simulink model "plantmodel"  (R2020a)
settings: Solver=VariableStepAuto  StartTime=0.0  StopTime=10.0  RelTol=1e-3
undefined symbols (not defined in the file): Ax, Ay, Az, b, d, g, I, Ixx, Iyy, Izz, Jr, m
settings Model: Creator=Muni Kumar  LastModifiedBy=Muni Kumar

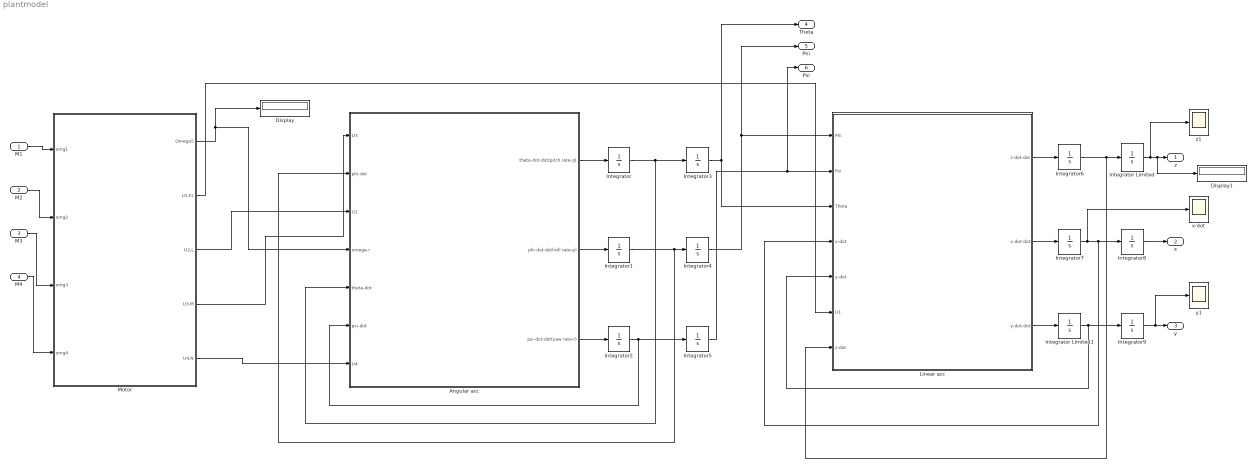
== system plantmodel ==
  M1 : Inport
  M2 : Inport  Port=2
  M3 : Inport  Port=3
  M4 : Inport  Port=4
  Angular acc : Subsystem
  Display : Display
      settings: Decimation=2
  Display1 : Display
  Integrator{,1..2,6..9} (7 alike) : Integrator
  Integrator Limited : Integrator  LimitOutput=on  UpperSaturationLimit=1  LowerSaturationLimit=0
  Integrator Limited1 : Integrator  LimitOutput=on  UpperSaturationLimit=1  LowerSaturationLimit=0
  Integrator3 : Integrator  WrapState=on
  Integrator4 : Integrator  WrapState=on
  Integrator5 : Integrator  WrapState=on
  Linear acc : Subsystem
  Motor : Subsystem
  x-dot : Scope
  y1 : Scope
  z1 : Scope
  z : Outport
  x : Outport  Port=2
  y : Outport  Port=3
  Theta : Outport  Port=4
  Phi : Outport  Port=5
  Psi : Outport  Port=6
  wires:
  Linear acc/2(x-dot-dot) -> Integrator7/1
  Integrator6/1 -> Integrator Limited/1, Linear acc/7(z-dot)
  Linear acc/1(z-dot-dot) -> Integrator6/1
  Motor/2(U1,Fz) -> Linear acc/6(U1)
  Linear acc/3(y-dot-dot) -> Integrator Limited1/1
  Integrator Limited1/1 -> Integrator9/1, Linear acc/5(y-dot)
  M3/1 -> Motor/3(omg3)
  M2/1 -> Motor/2(omg2)
  M1/1 -> Motor/1(omg1)
  M4/1 -> Motor/4(omg4)
  Angular acc/2(phi-dot-dot(roll rate-p)) -> Integrator1/1
  Angular acc/3(psi-dot-dot(yaw rate-r)) -> Integrator2/1
  Integrator/1 -> Angular acc/5(theta-dot), Integrator3/1
  Angular acc/1(theta-dot-dot(pitch rate-q)) -> Integrator/1
  Motor/5(U4,N) -> Angular acc/7(U4)
  Motor/4(U3,M) -> Angular acc/1(U3)
  Motor/3(U2,L) -> Angular acc/3(U2)
  Integrator1/1 -> Angular acc/2(phi-dot), Integrator4/1
  Integrator2/1 -> Angular acc/6(psi-dot), Integrator5/1
  Motor/1(Omega5) -> Display/1, Angular acc/4(omega-r)
  Integrator3/1 -> Linear acc/3(Theta), Theta/1
  Integrator4/1 -> Phi/1, Linear acc/1(Phi)
  Integrator5/1 -> Psi/1, Linear acc/2(Psi)
  Integrator Limited/1 -> z1/1, Display1/1, z/1
  Integrator8/1 -> x/1
  Integrator7/1 -> x-dot/1, Linear acc/4(x-dot), Integrator8/1
  Integrator9/1 -> y1/1, y/1

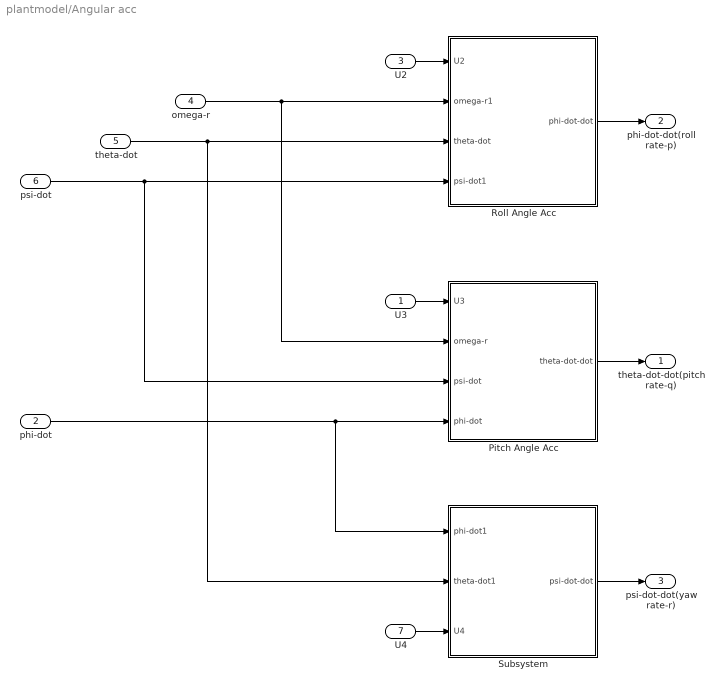
== system plantmodel/Angular acc ==
  U3 : Inport
  phi-dot : Inport  Port=2
  U2 : Inport  Port=3
  omega-r : Inport  Port=4
  theta-dot : Inport  Port=5
  psi-dot : Inport  Port=6
  U4 : Inport  Port=7
  Pitch Angle Acc : Subsystem
  Roll Angle Acc : Subsystem
  Subsystem : Subsystem
  theta-dot-dot(pitch rate-q) : Outport
  phi-dot-dot(roll rate-p) : Outport  Port=2
  psi-dot-dot(yaw rate-r) : Outport  Port=3
  wires:
  phi-dot/1 -> Subsystem/1(phi-dot1), Pitch Angle Acc/4(phi-dot)
  U2/1 -> Roll Angle Acc/1(U2)
  Roll Angle Acc/1(phi-dot-dot) -> phi-dot-dot(roll rate-p)/1
  U4/1 -> Subsystem/3(U4)
  theta-dot/1 -> Subsystem/2(theta-dot1), Roll Angle Acc/3(theta-dot)
  Subsystem/1(psi-dot-dot) -> psi-dot-dot(yaw rate-r)/1
  psi-dot/1 -> Pitch Angle Acc/3(psi-dot), Roll Angle Acc/4(psi-dot1)
  Pitch Angle Acc/1(theta-dot-dot) -> theta-dot-dot(pitch rate-q)/1
  U3/1 -> Pitch Angle Acc/1(U3)
  omega-r/1 -> Pitch Angle Acc/2(omega-r), Roll Angle Acc/2(omega-r1)

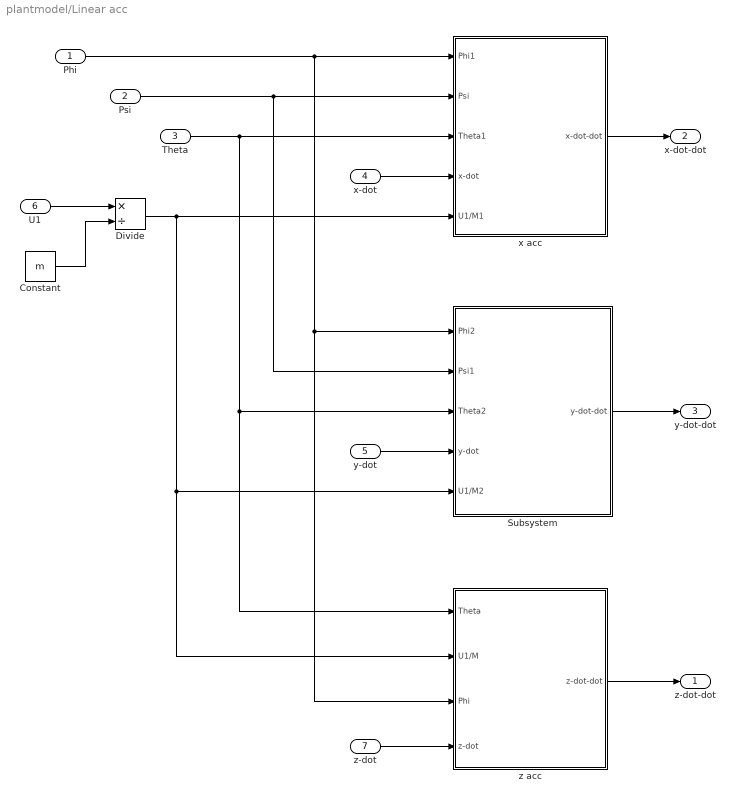
== system plantmodel/Linear acc ==
  Phi : Inport
  Psi : Inport  Port=2
  Theta : Inport  Port=3
  x-dot : Inport  Port=4
  y-dot : Inport  Port=5
  U1 : Inport  Port=6
  z-dot : Inport  Port=7
  Constant : Constant  Value=m
  Divide : Product  Inputs=*/
  Subsystem : Subsystem
  x acc : Subsystem
  z acc : Subsystem
  z-dot-dot : Outport
  x-dot-dot : Outport  Port=2
  y-dot-dot : Outport  Port=3
  wires:
  Theta/1 -> x acc/3(Theta1), Subsystem/3(Theta2), z acc/1(Theta)
  Phi/1 -> Subsystem/1(Phi2), z acc/3(Phi), x acc/1(Phi1)
  Divide/1 -> Subsystem/5(U1/M2), z acc/2(U1/M), x acc/5(U1/M1)
  y-dot/1 -> Subsystem/4(y-dot)
  Constant/1 -> Divide/2
  Psi/1 -> Subsystem/2(Psi1), x acc/2(Psi)
  z-dot/1 -> z acc/4(z-dot)
  U1/1 -> Divide/1
  x-dot/1 -> x acc/4(x-dot)
  x acc/1(x-dot-dot) -> x-dot-dot/1
  z acc/1(z-dot-dot) -> z-dot-dot/1
  Subsystem/1(y-dot-dot) -> y-dot-dot/1

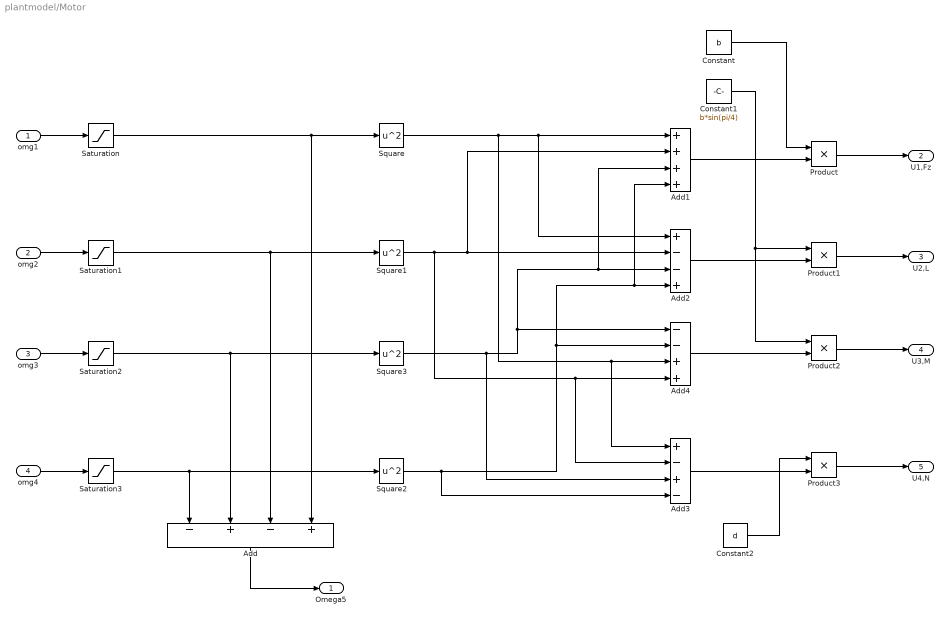
== system plantmodel/Motor ==
  omg1 : Inport
  omg2 : Inport  Port=2
  omg3 : Inport  Port=3
  omg4 : Inport  Port=4
  Add : Sum  Inputs=-+-+
  Add1 : Sum  Inputs=++++
  Add2 : Sum  Inputs=+--+
  Add3 : Sum  Inputs=+-+-
  Add4 : Sum  Inputs=--++
  Constant : Constant  Value=b
  Constant1 : Constant  Value=b*sin(pi/4)
  Constant2 : Constant  Value=d
  Product{,1..3} (4 alike) : Product
  Saturation{,1..3} (4 alike) : Saturate
  Square{,1..3} (4 alike) : Math  Operator=square  SaturateOnIntegerOverflow=on
  Omega5 : Outport
  U1,Fz : Outport  Port=2
  U2,L : Outport  Port=3
  U3,M : Outport  Port=4
  U4,N : Outport  Port=5
  wires:
  Product3/1 -> U4,N/1
  omg1/1 -> Saturation/1
  omg2/1 -> Saturation1/1
  Add/1 -> Omega5/1
  omg3/1 -> Saturation2/1
  Product2/1 -> U3,M/1
  Saturation/1 -> Add/4, Square/1
  Product1/1 -> U2,L/1
  Product/1 -> U1,Fz/1
  Add2/1 -> Product1/2
  Square3/1 -> Add3/3, Add4/1, Add1/3, Add2/3
  Square2/1 -> Add4/2, Add1/4, Add2/4, Add3/4
  Square/1 -> Add3/1, Add4/3, Add2/1, Add1/1
  Saturation3/1 -> Add/1, Square2/1
  Constant/1 -> Product/1
  Square1/1 -> Add3/2, Add4/4, Add1/2, Add2/2
  omg4/1 -> Saturation3/1
  Constant1/1 -> Product2/1, Product1/1
  Add4/1 -> Product2/2
  Add1/1 -> Product/2
  Add3/1 -> Product3/2
  Saturation2/1 -> Add/2, Square3/1
  Saturation1/1 -> Add/3, Square1/1
  Constant2/1 -> Product3/1

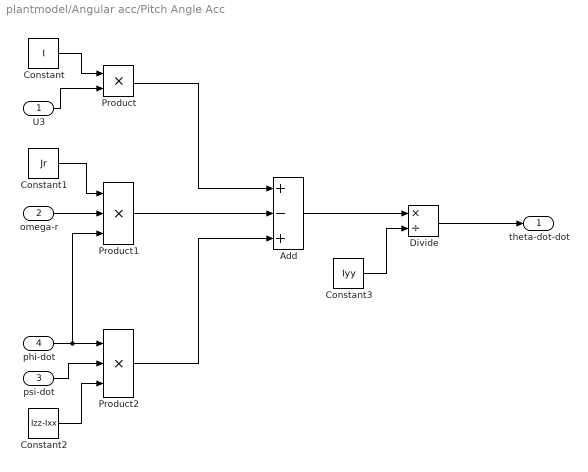
== system plantmodel/Angular acc/Pitch Angle Acc ==
  U3 : Inport
  omega-r : Inport  Port=2
  psi-dot : Inport  Port=3
  phi-dot : Inport  Port=4
  Add : Sum  Inputs=+-+
  Constant : Constant  Value=I
  Constant1 : Constant  Value=Jr
  Constant2 : Constant  Value=Izz-Ixx
  Constant3 : Constant  Value=Iyy
  Divide : Product  Inputs=*/
  Product : Product
  Product1 : Product  Inputs=3
  Product2 : Product  Inputs=3
  theta-dot-dot : Outport
  wires:
  Divide/1 -> theta-dot-dot/1
  Product/1 -> Add/1
  phi-dot/1 -> Product1/3, Product2/1
  psi-dot/1 -> Product2/2
  Product1/1 -> Add/2
  Constant1/1 -> Product1/1
  U3/1 -> Product/2
  Constant/1 -> Product/1
  Constant3/1 -> Divide/2
  Constant2/1 -> Product2/3
  omega-r/1 -> Product1/2
  Add/1 -> Divide/1
  Product2/1 -> Add/3

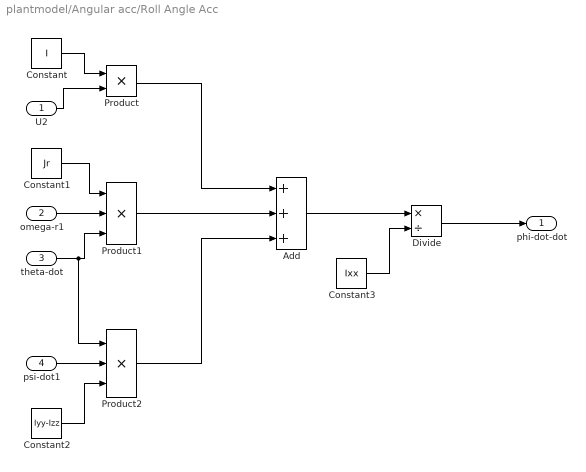
== system plantmodel/Angular acc/Roll Angle Acc ==
  U2 : Inport
  omega-r1 : Inport  Port=2
  theta-dot : Inport  Port=3
  psi-dot1 : Inport  Port=4
  Add : Sum  Inputs=+++
  Constant : Constant  Value=I
  Constant1 : Constant  Value=Jr
  Constant2 : Constant  Value=Iyy-Izz
  Constant3 : Constant  Value=Ixx
  Divide : Product  Inputs=*/
  Product : Product
  Product1 : Product  Inputs=3
  Product2 : Product  Inputs=3
  phi-dot-dot : Outport
  wires:
  psi-dot1/1 -> Product2/2
  Product/1 -> Add/1
  Constant/1 -> Product/1
  theta-dot/1 -> Product2/1, Product1/3
  Product1/1 -> Add/2
  Constant3/1 -> Divide/2
  Add/1 -> Divide/1
  Constant2/1 -> Product2/3
  Product2/1 -> Add/3
  U2/1 -> Product/2
  omega-r1/1 -> Product1/2
  Constant1/1 -> Product1/1
  Divide/1 -> phi-dot-dot/1

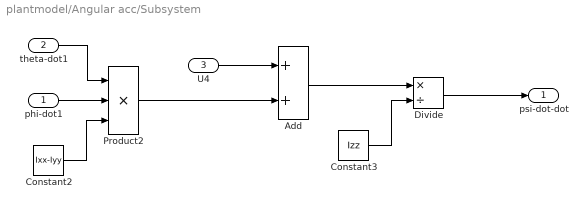
== system plantmodel/Angular acc/Subsystem ==
  phi-dot1 : Inport
  theta-dot1 : Inport  Port=2
  U4 : Inport  Port=3
  Add : Sum
  Constant2 : Constant  Value=Ixx-Iyy
  Constant3 : Constant  Value=Izz
  Divide : Product  Inputs=*/
  Product2 : Product  Inputs=3
  psi-dot-dot : Outport
  wires:
  Constant2/1 -> Product2/3
  phi-dot1/1 -> Product2/2
  Product2/1 -> Add/2
  theta-dot1/1 -> Product2/1
  Constant3/1 -> Divide/2
  Add/1 -> Divide/1
  U4/1 -> Add/1
  Divide/1 -> psi-dot-dot/1

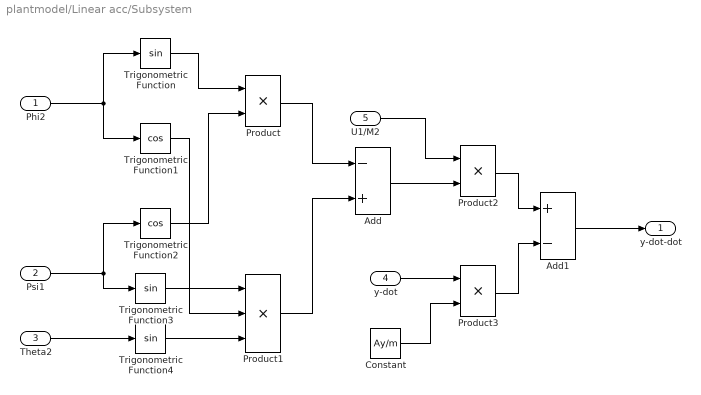
== system plantmodel/Linear acc/Subsystem ==
  Phi2 : Inport
  Psi1 : Inport  Port=2
  Theta2 : Inport  Port=3
  y-dot : Inport  Port=4
  U1/M2 : Inport  Port=5
  Add : Sum  Inputs=-+
  Add1 : Sum  Inputs=+-
  Constant : Constant  Value=Ay/m
  Product : Product
  Product1 : Product  Inputs=3
  Product2 : Product
  Product3 : Product
  Trigonometric Function : Trigonometry
  Trigonometric Function1 : Trigonometry  Operator=cos
  Trigonometric Function2 : Trigonometry  Operator=cos
  Trigonometric Function3 : Trigonometry
  Trigonometric Function4 : Trigonometry
  y-dot-dot : Outport
  wires:
  Phi2/1 -> Trigonometric Function1/1, Trigonometric Function/1
  Theta2/1 -> Trigonometric Function4/1
  Trigonometric Function1/1 -> Product1/2
  Add1/1 -> y-dot-dot/1
  Psi1/1 -> Trigonometric Function3/1, Trigonometric Function2/1
  Trigonometric Function4/1 -> Product1/3
  y-dot/1 -> Product3/1
  Product2/1 -> Add1/1
  U1/M2/1 -> Product2/1
  Product1/1 -> Add/2
  Add/1 -> Product2/2
  Constant/1 -> Product3/2
  Product/1 -> Add/1
  Trigonometric Function3/1 -> Product1/1
  Product3/1 -> Add1/2
  Trigonometric Function/1 -> Product/1
  Trigonometric Function2/1 -> Product/2

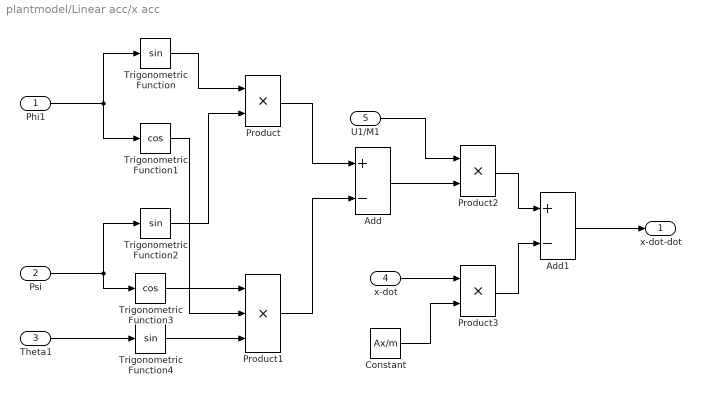
== system plantmodel/Linear acc/x acc ==
  Phi1 : Inport
  Psi : Inport  Port=2
  Theta1 : Inport  Port=3
  x-dot : Inport  Port=4
  U1/M1 : Inport  Port=5
  Add : Sum  Inputs=+-
  Add1 : Sum  Inputs=+-
  Constant : Constant  Value=Ax/m
  Product : Product
  Product1 : Product  Inputs=3
  Product2 : Product
  Product3 : Product
  Trigonometric Function : Trigonometry
  Trigonometric Function1 : Trigonometry  Operator=cos
  Trigonometric Function2 : Trigonometry
  Trigonometric Function3 : Trigonometry  Operator=cos
  Trigonometric Function4 : Trigonometry
  x-dot-dot : Outport
  wires:
  Phi1/1 -> Trigonometric Function1/1, Trigonometric Function/1
  x-dot/1 -> Product3/1
  Product3/1 -> Add1/2
  U1/M1/1 -> Product2/1
  Psi/1 -> Trigonometric Function3/1, Trigonometric Function2/1
  Trigonometric Function3/1 -> Product1/1
  Theta1/1 -> Trigonometric Function4/1
  Add/1 -> Product2/2
  Trigonometric Function1/1 -> Product1/2
  Trigonometric Function2/1 -> Product/2
  Product1/1 -> Add/2
  Product2/1 -> Add1/1
  Trigonometric Function/1 -> Product/1
  Trigonometric Function4/1 -> Product1/3
  Product/1 -> Add/1
  Constant/1 -> Product3/2
  Add1/1 -> x-dot-dot/1

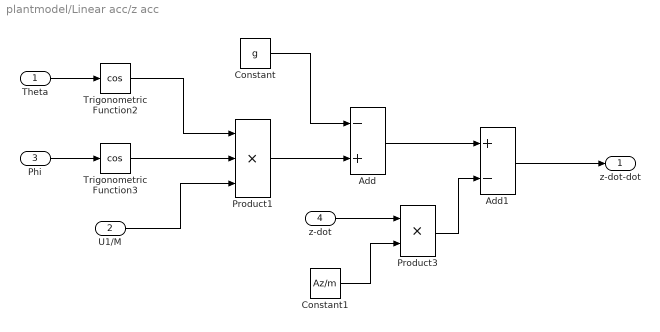
== system plantmodel/Linear acc/z acc ==
  Theta : Inport
  U1/M : Inport  Port=2
  Phi : Inport  Port=3
  z-dot : Inport  Port=4
  Add : Sum  Inputs=-+
  Add1 : Sum  Inputs=+-
  Constant : Constant  Value=g
  Constant1 : Constant  Value=Az/m
  Product1 : Product  Inputs=3
  Product3 : Product
  Trigonometric Function2 : Trigonometry  Operator=cos
  Trigonometric Function3 : Trigonometry  Operator=cos
  z-dot-dot : Outport
  wires:
  Phi/1 -> Trigonometric Function3/1
  Product3/1 -> Add1/2
  U1/M/1 -> Product1/3
  Theta/1 -> Trigonometric Function2/1
  Add/1 -> Add1/1
  Product1/1 -> Add/2
  Add1/1 -> z-dot-dot/1
  Constant1/1 -> Product3/2
  z-dot/1 -> Product3/1
  Trigonometric Function3/1 -> Product1/2
  Constant/1 -> Add/1
  Trigonometric Function2/1 -> Product1/1
